simulink model "P_CGMRES_slow"  (R2023a)
settings: Solver=FixedStepAuto  StartTime=0.0  StopTime=22.5  RelTol=1e-3
values from neighbouring files (symbols this model uses):
  lujing = 8    [main.m]
libraries: Solver_SF x1
(part 16 of 21)

== matlab function P_CGMRES_slow/单车道避障参考坐标/纵向滑移量计算模块1 ==
  data: target input; y output
function y  = fcn(target)
y_global=[0	0	0	0	0	0	0	0	0	0	0	0	0	0	0	0	0	0	0	0	0	0	0	0	0	0	0	0	0	0	0	0	0	0	0	0	0	0	0	0	0	0	0	0	0	0	0	0	0	0	0	0	0	0	0	0	0	0	0	0	0	0	0	0	0	0	0	0	0	0	0	0	0	0	0	0	0	0	0	0	0	0	0	0	0	0	0	0	0	0	0	0	0	0	0	0	0	0	0	0	0	0	0	0	0	0	0	0	0	0	0	0	0	0	0	0	0	0	0	0	0	0	0	0	0	0	0	0	0	0	0	0	0	0	0	0	0	0	0	0	0	0	0	0	0	0	0	0	0	0	0	0	0	0	0	0	0	0	0	0	0	0	0	0	0	0	0	0	0	0	0	0	0	0	0	0	0	0	0	0	0	0	0	0	0	0	0	0	0	0	0	0	0	0	0	0	0	0	0	0	0	0	0	0	0	0	0	0	0	0	0	0	0	0	0	0	0	0	0	0	0	0	0	0	0	0	0	0	0	0	0	0	0	0	0	0	0	0	0	0	0	0	0	0	0	0	0	0	0	0	0	0	0	0	0	0	0	0	0	0	0	0	0	0	0	0	0	0	0	0	0	0	0	0	0	0	0	0	0	0	0	0	0	0	0	0	0	0	0	0	0	0	0	0	0	0	0	0	0	0	0	0	0	0	0	0	0	0	0	0	0	0	0	0	0	0	0	0	0	0	0	0	0	0	0	0	0	0	0	0	0	0	0	0	0	0	0	0	0	0	0	0	0	0	0	0	0	0	0	0	0	0	0	0	0	0	0	0	0	0	0	0	0	0	0	0	0	0	0	0	0	0	0	0	0	0	0	0	0	0	0	0	0	0	0	0	0	0	0	0	0	0	0	0	0	0	0	0	0	0	0	0	0	0	0	0	0	0	0	0	0	0	0	0	0	0	0	0	0	0	0	0	0	0	0	0	0	0	0	0	0	0	0	0	0	0	0	0	0	0	0	0	0	0	0	0	0	0	0	0	0	0	0	0	0	0	0	0	0	0	0	0	0	0	0	0	0	0	0	0	0	0	0	0	0	0	0	0	0	0	0	0	0	0	0	0	0	0	0	0	0	0	0	0	0	0	0	0	0	0];
y=0;
if target>length(y_global)-10
    y=1;
end

== matlab function P_CGMRES_slow/单车道障碍车位置/障碍车1位置 ==
  data: x_obs output; y_obs output; t input
function [x_obs,y_obs] = fcn(t)
N=7;
x_obs=50*ones(N,1);
y_obs=0*ones(N,1);
if t>1
    x_obs=50+10*(t-1)*ones(N,1);
    y_obs=0*ones(N,1);
end

if t>1
    x_obs=50+10*(t-1)*ones(N,1);
    y_obs=0*ones(N,1);
end

== matlab function P_CGMRES_slow/单车道障碍车位置/障碍车1位置1 ==
  data: x_obs output; y_obs output; t input
function [x_obs,y_obs] = fcn(t)
x_obs=120;
y_obs=1;
if t>1
    x_obs=120+10*(t-1);
    y_obs=1;
end
